simulink model "FirstCode_SoftwareHarness"  (R2014b)
settings: Solver=FixedStepDiscrete  StartTime=0.0  StopTime=10  RelTol=1e-3
PostLoadFcn:
  | c2000demoscallback(1)
undefined symbols (not defined in the file or in its folder): CR, serial
libraries: instrumentlib x3
settings Model: Creator=The MathWorks Inc.  LastModifiedBy=Nathan
settings DataIOCC: SignalLoggingSaveFormat=ModelDataLogs  SaveOutput=off  SaveTime=off
settings OptimizationCC: ExpressionDepthLimit=2147483647  InitFltsAndDblsToZero=on  OptimizeModelRefInitCode=on  LifeSpan=Inf  MaxStackSize=64
settings DebuggingCC: UnderspecifiedInitializationDetection=Classic  MergeDetectMultiDrivingBlocksExec=none  SignalResolutionControl=TryResolveAllWithWarning  SolverPrmCheckMsg=none  InheritedTsInSrcMsg=none  MultiTaskDSMMsg=warning  MultiTaskCondExecSysMsg=none  FcnCallInpInsideContextMsg=UseLocalSettings  StateNameClashWarn=warning
settings HardwareCC: ProdBitPerChar=16  ProdBitPerInt=16  ProdBitPerPointer=16  ProdLargestAtomicInteger=Integer  ProdIntDivRoundTo=Zero  ProdEndianess=LittleEndian  ProdWordSize=16  ProdHWDeviceType=Texas Instruments->C2000  TargetBitPerChar=16  TargetBitPerInt=16  TargetBitPerPointer=16  TargetLargestAtomicInteger=Integer  TargetIntDivRoundTo=Zero  TargetEndianess=LittleEndian  TargetWordSize=16  TargetHWDeviceType=Texas Instruments->C2000
settings RTWCC: SystemTargetFile=ert.tlc  TemplateMakefile=ert_default_tmf  PostCodeGenCommand=; ;codertarget.postCodeGenHookCommand(h)  Description=Embedded Coder  GenerateReport=on  ProcessScript=ert_make_rtw_hook  Toolchain=Texas Instruments Code Composer Studio v5 (C2000)  BuildConfiguration=Faster Runs  IncludeHyperlinkInReport=on  PortableWordSizes=on  CodeExecutionProfiling=on  CodeProfilingInstrumentation=on
settings CodeAppCC: IgnoreCustomStorageClasses=off  CustomSymbolStrType=$N$R$M  InternalIdentifier=Classic

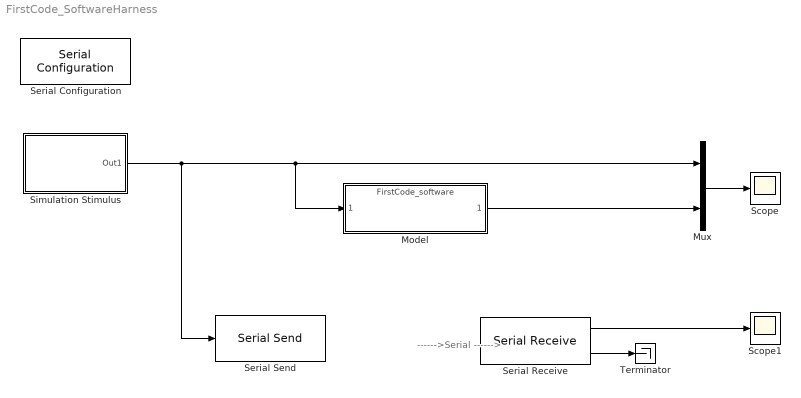
== system FirstCode_SoftwareHarness ==
  note: ------>Serial ------>
  Model : ModelReference  ModelNameDialog=FirstCode_software.slx  SimulationMode=Normal  ModelReferenceVersion=1.83  CopyOfModelName=FirstCode_software.slx  DefaultDataLogging=on
  Mux : Mux  Inputs=2
  Scope : Scope
  Scope1 : Scope
  Serial Configuration : instrumentlib/Serial Configuration  Priority=-200000  ComPortMenu=<Please select a port...>  ComPort=COM11  ObjConstructor=serial('COM11');  BaudRate=9600  DataBits=8  Parity=none  StopBits=1  FlowControl=none  Timeout=10  ByteOrder=LittleEndian
  Serial Receive : instrumentlib/Serial Receive  ComPortMenu=COM11  ComPort=COM11  ObjConstructor=serial('COM11');  Terminator=<none>  DataSize=[1 1]  DataType=uint8  EnableBlockingMode=off  ActionDataUnavailable=Output last received value  CustomValue=0  SampleTime=0.01
  Serial Send : instrumentlib/Serial Send  ComPortMenu=<Please select a port...>  ComPort=COM11  ObjConstructor=serial('COM11');  Header='S'  Terminator=CR ('\r')  EnableBlockingMode=on
  Simulation Stimulus : Subsystem
  Terminator : Terminator
  wires:
  Simulation Stimulus/1(Out1) -> Serial Send/1, Model/1, Mux/1
  Mux/1 -> Scope/1
  Model/1 -> Mux/2
  Serial Receive/1 -> Scope1/1
  Serial Receive/2 -> Terminator/1

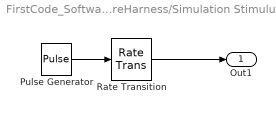
== system FirstCode_SoftwareHarness/Simulation Stimulus ==
  Pulse Generator : DiscretePulseGenerator  PulseType=Time based  Period=1  PulseWidth=50
  Rate Transition : RateTransition  OutPortSampleTime=0.1
  Out1 : Outport
  wires:
  Pulse Generator/1 -> Rate Transition/1
  Rate Transition/1 -> Out1/1
